simulink model "Model_M3"  (R2018a)
settings: Solver=VariableStepAuto  StartTime=0.0  StopTime=50
libraries: simulink x3
settings Model: Creator=Aniket Raj  LastModifiedBy=Aniket Raj
settings SolverCC: MaxConsecutiveMinStep=5

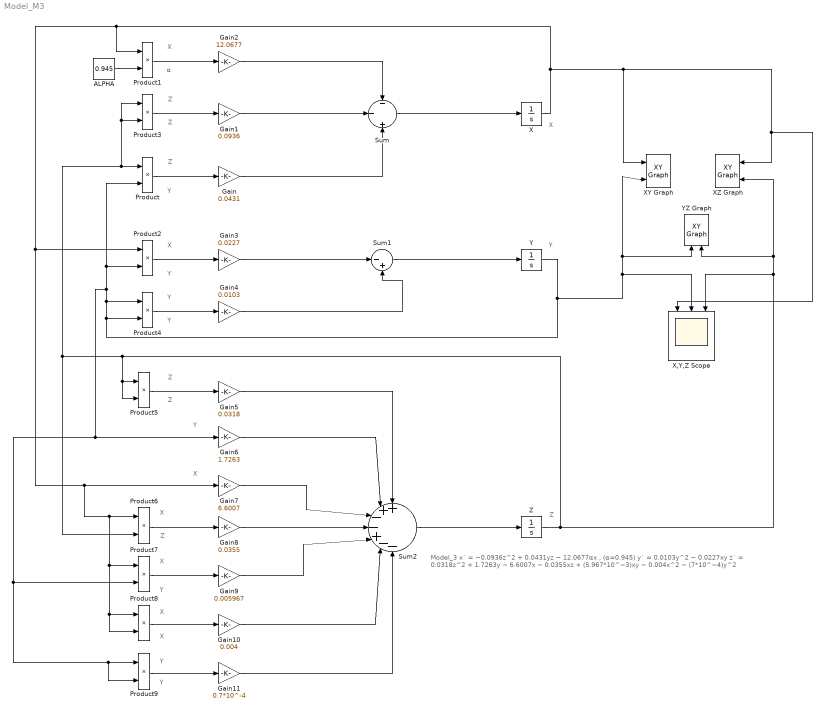
== system Model_M3 ==
  note: Model_3
      |
      | x˙ = −0.0936z^2 + 0.0431yz − 12.0677αx , (α=0.945)
      | y˙ = 0.0103y^2 − 0.0227xy
      | z˙ = 0.0318z^2 + 1.7263y − 6.6007x − 0.0355xz + (5.967*10^−3)xy − 0.004x^2 − (7*10^−4)y^2
  note: X
  note: Y
  note: Z
  note: Z
  note: Y
  note: Z
  note: X
  note: X
  note: Y
  note: Y
  note: Z
  note: Y
  note: X
  note: X
  note: Z
  note: Y
  note: X
  note: Y
  note: X
  note: Z
  note: Y
  note: Z
  note: X
  note: Y
  note: α
  ALPHA : Constant  Value=0.945
  Gain : Gain  Gain=0.0431
  Gain1 : Gain  Gain=0.0936
  Gain10 : Gain  Gain=0.004
  Gain11 : Gain  Gain=0.7*10^-4
  Gain2 : Gain  Gain=12.0677
  Gain3 : Gain  Gain=0.0227
  Gain4 : Gain  Gain=0.0103
  Gain5 : Gain  Gain=0.0318
  Gain6 : Gain  Gain=1.7263
  Gain7 : Gain  Gain=6.6007
  Gain8 : Gain  Gain=0.0355
  Gain9 : Gain  Gain=0.005967
  Product{,1..9} (10 alike) : Product
  Sum : Sum  Inputs=-|-|+
  Sum1 : Sum  Inputs=|-+
  Sum2 : Sum  Inputs=+|+|-|-|+|-|-
  X : Integrator  InitialCondition=344.0896
  X,Y,Z Scope : Scope  NumInputPorts=3
  "XY Graph " : simulink/Sinks/XY Graph  Tag=XY GRAPH  xmin=-500  xmax=3000  ymin=-500  ymax=5000  st=0.01
  XZ Graph : simulink/Sinks/XY Graph  xmin=-200  xmax=3000  ymin=-200  ymax=1000  st=0.01
  Y : Integrator  InitialCondition=627.7882
  YZ Graph : simulink/Sinks/XY Graph  xmin=-500  xmax=4000  ymin=-500  ymax=500  st=0.01
  Z : Integrator  InitialCondition=101.5058
  wires:
  Sum/1 -> X/1
  Sum1/1 -> Y/1
  Sum2/1 -> Z/1
  Gain/1 -> Sum/3
  Product/1 -> Gain/1
  Product3/1 -> Gain1/1
  Gain1/1 -> Sum/2
  Product2/1 -> Gain3/1
  Gain3/1 -> Sum1/1
  Product4/1 -> Gain4/1
  Gain4/1 -> Sum1/2
  Product5/1 -> Gain5/1
  Gain5/1 -> Sum2/1
  Gain6/1 -> Sum2/2
  Gain7/1 -> Sum2/3
  Product6/1 -> Gain8/1
  Gain8/1 -> Sum2/4
  Product7/1 -> Gain9/1
  Gain9/1 -> Sum2/5
  Product8/1 -> Gain10/1
  Gain10/1 -> Sum2/6
  Product9/1 -> Gain11/1
  Gain11/1 -> Sum2/7
  Z/1 -> Product3/1, Product3/2, Product/1, Product6/2, Product5/2, Product5/1, X,Y,Z Scope/3, XZ Graph/2, YZ Graph/2
  ALPHA/1 -> Product1/2
  Product1/1 -> Gain2/1
  Gain2/1 -> Sum/1
  Y/1 -> Product4/1, Product9/2, Product9/1, Product7/2, Gain6/1, Product2/2, Product/2, Product4/2, X,Y,Z Scope/2, "XY Graph "/2, YZ Graph/1
  X/1 -> "XY Graph "/1, XZ Graph/1, X,Y,Z Scope/1, Product1/1, Product8/2, Product8/1, Product7/1, Product6/1, Gain7/1, Product2/1
